simulink model "control_nivel"  (R2018b)
settings: Solver=VariableStepAuto  StartTime=0.0  StopTime=Inf  FixedStep=0.3  RelTol=1e-2
StopFcn:
  | fileName=['dateSimulare_',sprintf('%d',nr_simulare),'.mat'];
  | save(fileName,'simulink_referintaDebit','simulink_referintaNivel1','simulink_referintaNivel2','simulink_comandaPompa','simulink_comandaServo1','simulink_comandaServo2','simulink_debit1','simulink_debit2','simulink_debit3','simulink_nivel1','simulink_nivel2');
  | nr_simulare=nr_simulare+1;
undefined symbols (not defined in the file or in its folder): Hr_debit_d
libraries: sldrtlib x1
settings Model: Creator=Elena  LastModifiedBy=Elena

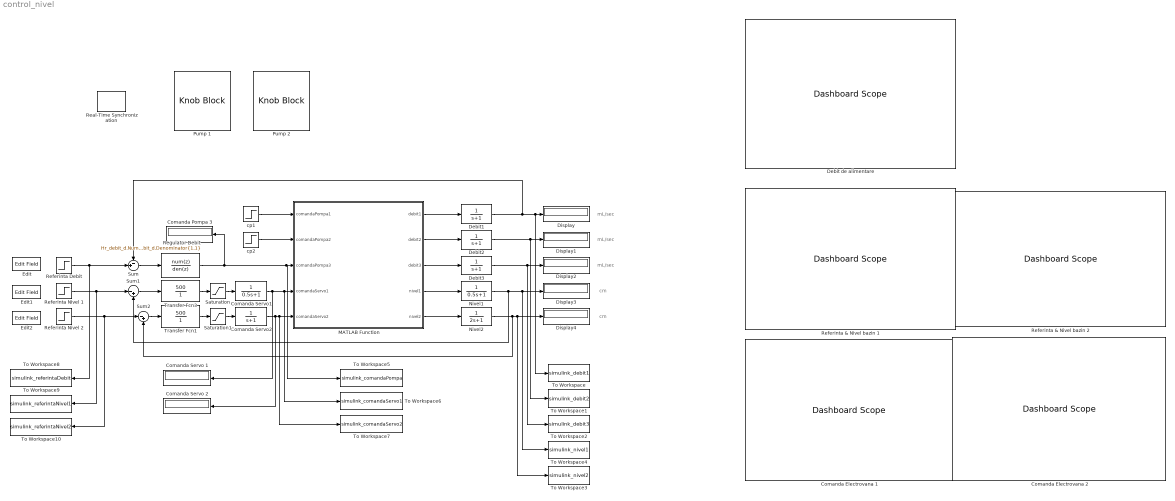
== system control_nivel ==
  note: mL/sec
  note: mL/sec
  note: mL/sec
  note: cm
  note: cm
  Comanda Electrovana 1 : DashboardScope  WebBlockId=154  TimeSpan=600  Ymin=0  Ymax=110
  Comanda Electrovana 2 : DashboardScope  WebBlockId=155  TimeSpan=600  Ymin=0  Ymax=110
  Comanda Pompa 3 : Display
  Comanda Servo 1 : Display
  Comanda Servo 2 : Display
  Comanda Servo1 : TransferFcn  Denominator=[0.5 1]
  Comanda Servo2 : TransferFcn  Denominator=[1 1]
  Debit de alimentare : DashboardScope  WebBlockId=153  TimeSpan=600  Ymin=0  Ymax=17
  Debit1 : TransferFcn  Denominator=[1 1]
  Debit2 : TransferFcn  Denominator=[1 1]
  Debit3 : TransferFcn  Denominator=[1 1]
  Display{,1..4} (5 alike) : Display
      Display settings: Format=short_e
      Display1 settings: Format=short_e
      Display2 settings: Format=short_e
  Edit : EditField  WebBlockId=61  LabelPosition=Hide  ShowInitialText=on  Alignment=Center
  Edit1 : EditField  WebBlockId=85  LabelPosition=Hide  ShowInitialText=on  Alignment=Center
  Edit2 : EditField  WebBlockId=86  LabelPosition=Hide  ShowInitialText=on  Alignment=Center
  MATLAB Function : MATLAB Function  TreatAsAtomicUnit=on  SystemSampleTime=0.3
  Nivel1 : TransferFcn  Denominator=[0.5 1]
  Nivel2 : TransferFcn  Denominator=[2 1]
  "Pump 1 " : KnobBlock  WebBlockId=13  LabelPosition=Hide  TickInterval=10
  Pump 2 : KnobBlock  WebBlockId=27  LabelPosition=Hide  TickInterval=10
  Real-Time Synchronization : sldrtlib/Real-Time Synchronization  SampleTime=0.3  MaxMissedTicks=100000  ShowMissedTicks=off  YieldWhenWaiting=on
  Referinta & Nivel bazin 1 : DashboardScope  WebBlockId=152  TimeSpan=600  Ymin=0  Ymax=15
  Referinta & Nivel bazin 2 : DashboardScope  WebBlockId=146  TimeSpan=600  Ymin=0  Ymax=15
  "Referinta Debit " : Step  Time=0  After=5  SampleTime=0.3
  "Referinta NIvel 1 " : Step  Time=0  After=2  SampleTime=0.3
  Referinta Nivel 2 : Step  Time=0  SampleTime=0.3
  Regulator Debit : DiscreteTransferFcn  Numerator=Hr_debit_d.Numerator{1,1}  Denominator=Hr_debit_d.Denominator{1,1}  SampleTime=0.3
  Saturation : Saturate  UpperLimit=100  LowerLimit=0
  Saturation1 : Saturate  UpperLimit=100  LowerLimit=0
  Sum : Sum  Inputs=-+|
  Sum1 : Sum  Inputs=|-+
  Sum2 : Sum  Inputs=|-+
  To Workspace : ToWorkspace  VariableName=simulink_debit1  SampleTime=0.3
      settings: Save2DSignal=2-D array (concatenate along first dimension)
  To Workspace1 : ToWorkspace  VariableName=simulink_debit2  SampleTime=0.3
      settings: Save2DSignal=2-D array (concatenate along first dimension)
  To Workspace10 : ToWorkspace  VariableName=simulink_referintaNivel2  SampleTime=0.3
      settings: Save2DSignal=2-D array (concatenate along first dimension)
  To Workspace2 : ToWorkspace  VariableName=simulink_debit3  SampleTime=0.3
      settings: Save2DSignal=2-D array (concatenate along first dimension)
  To Workspace3 : ToWorkspace  VariableName=simulink_nivel2  SampleTime=0.3
      settings: Save2DSignal=2-D array (concatenate along first dimension)
  To Workspace4 : ToWorkspace  VariableName=simulink_nivel1  SampleTime=0.3
      settings: Save2DSignal=2-D array (concatenate along first dimension)
  To Workspace5 : ToWorkspace  VariableName=simulink_comandaPompa  SampleTime=0.3
      settings: Save2DSignal=2-D array (concatenate along first dimension)
  To Workspace6 : ToWorkspace  VariableName=simulink_comandaServo1  SampleTime=0.3
      settings: Save2DSignal=2-D array (concatenate along first dimension)
  To Workspace7 : ToWorkspace  VariableName=simulink_comandaServo2  SampleTime=0.3
      settings: Save2DSignal=2-D array (concatenate along first dimension)
  To Workspace8 : ToWorkspace  VariableName=simulink_referintaDebit  SampleTime=0.3
      settings: Save2DSignal=2-D array (concatenate along first dimension)
  To Workspace9 : ToWorkspace  VariableName=simulink_referintaNivel1  SampleTime=0.3
      settings: Save2DSignal=2-D array (concatenate along first dimension)
  Transfer Fcn1 : TransferFcn  Numerator=[500]  Denominator=[1]
  Transfer Fcn3 : TransferFcn  Numerator=[500]  Denominator=[1]
  cp1 : Step  Time=0  After=100  SampleTime=0
  cp2 : Step  Time=0  After=100  SampleTime=0
  wires:
  cp1/1 -> MATLAB Function/1(comandaPompa1)
  cp2/1 -> MATLAB Function/2(comandaPompa2)
  Debit1/1 -> Sum/1, To Workspace/1, Display/1
  MATLAB Function/1(debit1) -> Debit1/1
  "Referinta Debit "/1 -> To Workspace8/1, Sum/2
  Sum/1 -> Regulator Debit/1
  Debit2/1 -> To Workspace1/1, Display1/1
  MATLAB Function/2(debit2) -> Debit2/1
  MATLAB Function/3(debit3) -> Debit3/1
  Debit3/1 -> To Workspace2/1, Display2/1
  Regulator Debit/1 -> To Workspace5/1, MATLAB Function/3(comandaPompa3), Comanda Pompa 3/1
  MATLAB Function/4(nivel1) -> Nivel1/1
  Nivel1/1 -> To Workspace4/1, Display3/1, Sum1/2
  Nivel2/1 -> To Workspace3/1, Display4/1, Sum2/2
  MATLAB Function/5(nivel2) -> Nivel2/1
  "Referinta NIvel 1 "/1 -> To Workspace9/1, Sum1/1
  Sum1/1 -> Transfer Fcn3/1
  Transfer Fcn3/1 -> Saturation/1
  Saturation/1 -> Comanda Servo1/1
  Referinta Nivel 2/1 -> To Workspace10/1, Sum2/1
  Sum2/1 -> Transfer Fcn1/1
  Transfer Fcn1/1 -> Saturation1/1
  Saturation1/1 -> Comanda Servo2/1
  Comanda Servo1/1 -> To Workspace6/1, MATLAB Function/4(comandaServo1), Comanda Servo 1/1
  Comanda Servo2/1 -> To Workspace7/1, MATLAB Function/5(comandaServo2), Comanda Servo 2/1

== matlab function control_nivel/MATLAB Function ==
  data: comandaPompa1 input; debit1 output; comandaPompa2 input; comandaPompa3 input; comandaServo1 input; comandaServo2 input; debit2 output; debit3 output; nivel1 output; nivel2 output
function [debit1, debit2, debit3, nivel1, nivel2] = serialCommunication(comandaPompa1, comandaPompa2, comandaPompa3, comandaServo1, comandaServo2)

%     if not(exist('device', 'var'))
%         device = serial('COM6','BaudRate',115200);
%     end

%     fopen(device);

    coder.extrinsic('evalin')
    coder.extrinsic('fgets')
    coder.extrinsic('sscanf')
    
    debit1 = 0;
    debit2 = 0;
    debit3 = 0;
    nivel1 = 0;
    nivel2 = 0;
    
    device = evalin('base','device');
    
    fprintf(device, '%6.2f %6.2f %6.2f %6.2f %6.2f \n', [comandaPompa1 comandaPompa2 comandaPompa3 comandaServo1 comandaServo2]);
    receive = fgets(device)
    senzori = sscanf(receive, "%f")
    
    debit1 = senzori(1);
    debit2 = senzori(2);
    debit3 = senzori(3);
    nivel1 = senzori(4);
    nivel2 = senzori(5);

%      fclose(device);
end
